simulink model "success_0516_kjh_stair_test"  (R2022b)
settings: Solver=ode45  StartTime=0.0  StopTime=15  MaxStep=0.3  RelTol=1e-3
values from neighbouring files (symbols this model uses):
  g = 9.81    [make_circle.m]
undefined symbols (not defined in the file or in its folder): fifth, first, fourth, pane, second, third, X, Y, Z
libraries: sm_lib x151, nesl_utility x13, simulink x10, slpidlib x5, Contact_Forces_Lib x2
(part 6 of 6)

== system success_0516_kjh_stair_test/right wheel ==
  Cylindrical Solid4 : sm_lib/Body Elements/Cylindrical Solid  GraphicAmbientColor=[0.15 0.15 0.15 1.0]  BasedOnType=Mass  CenterOfMass=[0 0 0]  CenterOfMassUnits=m  GraphicDiffuseColor=[0.5 0.5 0.5]  CylinderLength=150  CylinderLengthUnits=mm  CylinderRadius=5  CylinderRadiusUnits=mm  Density=2700  DensityUnits=kg/m^3  DoExposeReferenceFrame=on  GraphicEmissiveColor=[0.0 0.0 0.0 1.0]  ExportEntireGeometry=on  SerializedFrames=<Frames/>  MarkerShape=Sphere  MarkerSize=10  GraphicType=FromGeometry  InertiaType=CalculateFromGeometry  Mass=115  MassUnits=g  MomentsOfInertia=[1 1 1]  MomentsOfInertiaUnits=kg*m^2  GraphicOpacity=1.0  ProductsOfInertia=[0 0 0]  ProductsOfInertiaUnits=kg*m^2  GraphicShininess=75  GraphicSpecularColor=[0.5 0.5 0.5 1.0]  GraphicVisPropType=SimpleVisualProperties
  File Solid1 : sm_lib/Body Elements/File Solid  ExtGeomFileName=C:\Users\vbnfg\OneDrive\바탕 화면\Castone design - 복사본\tyre_ipt_2dd205d0.STEP  UnitType=FromFile  ExtGeomFileUnits=m  StepReaderType=HEX  ExportConvexHullGeometry=on  InertiaType=CalculateFromGeometry  Mass=0.12  MassUnits=kg  CenterOfMass=[0 0 0]  CenterOfMassUnits=m  MomentsOfInertia=[1 1 1]  MomentsOfInertiaUnits=kg*m^2  ProductsOfInertia=[0 0 0]  ProductsOfInertiaUnits=kg*m^2  BasedOnType=Mass  Density=2700  DensityUnits=kg/m^3  DoExposeReferenceFrame=on  SerializedFrames=<Frames/>  GraphicType=FromGeometry  MarkerShape=Sphere  MarkerSize=10  GraphicVisPropType=SimpleVisualProperties  GraphicDiffuseColor=[0.5 0.5 0.5]  GraphicSpecularColor=[0.5 0.5 0.5 1.0]  GraphicAmbientColor=[0.15 0.15 0.15 1.0]  GraphicEmissiveColor=[0.0 0.0 0.0 1.0]  GraphicShininess=75  GraphicOpacity=1.0
  File Solid7 : sm_lib/Body Elements/File Solid  ExtGeomFileName=C:\Users\vbnfg\OneDrive\바탕 화면\Castone design - 복사본\wheel.stp  UnitType=FromFile  ExtGeomFileUnits=m  StepReaderType=HEX  ExportConvexHullGeometry=on  InertiaType=CalculateFromGeometry  Mass=1.2  MassUnits=kg  CenterOfMass=[0 0 0]  CenterOfMassUnits=m  MomentsOfInertia=[1 1 1]  MomentsOfInertiaUnits=kg*m^2  ProductsOfInertia=[0 0 0]  ProductsOfInertiaUnits=kg*m^2  BasedOnType=Mass  Density=2700  DensityUnits=kg/m^3  DoExposeReferenceFrame=on  SerializedFrames=<Frames/>  GraphicType=FromGeometry  MarkerShape=Sphere  MarkerSize=10  GraphicVisPropType=SimpleVisualProperties  GraphicDiffuseColor=[0.5 0.5 0.5]  GraphicSpecularColor=[0.5 0.5 0.5 1.0]  GraphicAmbientColor=[0.15 0.15 0.15 1.0]  GraphicEmissiveColor=[0.0 0.0 0.0 1.0]  GraphicShininess=75  GraphicOpacity=1.0
  Rigid Transform22 : sm_lib/Frames and Transforms/Rigid Transform  TranslationMethod=StandardAxis  TranslationStandardOffset=-50  TranslationLengthUnit=mm  TranslationStandardAxis=+Z  TranslationCartesianOffset=[0 0 -10]  TranslationROffset=0  TranslationROffsetUnits=m  TranslationZOffset=0  TranslationZOffsetUnits=m  TranslationThetaOffset=0  TranslationThetaOffsetUnits=deg  RotationMethod=None  RotationAngleUnits=deg  RotationStandardAxis=+Z  RotationAngle=0.0  RotationArbitraryAxis=[0 0 1]  FollAlignAxisA=+X  BaseAlignAxisA=+Y  FollAlignAxisB=+Y  BaseAlignAxisB=+Z  RotationSequenceAxes=FollowerAxes  RotationSequence=XYZ  RotationSequenceAngles=[0 90 -90]  RotationSequenceAnglesUnits=deg  RotationMatrix=[1 0 0; 0 1 0; 0 0 1]  Quaternion=[1 0 0 0]
  Conn1 : PMIOPort  Side=Left
  G2 : PMIOPort  Port=2  Side=Left
  G1 : PMIOPort  Port=3  Side=Left
  connections:
  Rigid Transform22/LConn1 -- Conn1/RConn1 -- Cylindrical Solid4/RConn1
  File Solid7/RConn1 -- File Solid1/RConn1 -- Rigid Transform22/RConn1
  Cylindrical Solid4/LConn1 -- G2/RConn1
  G1/RConn1 -- File Solid1/LConn1

== system success_0516_kjh_stair_test/추진블록 ==
  Ramp : simulink/Sources/Ramp  slope=-2  start=1  InitialOutput=0
  Ramp1 : simulink/Sources/Ramp  slope=2  start=2  InitialOutput=0
  Scope1 : Scope
  Sum1 : Sum  Inputs=|+++++++
  Out1 : Outport
  wires:
  Sum1/1 -> Out1/1, Scope1/1
  Ramp/1 -> Sum1/5
  Ramp1/1 -> Sum1/6

== system success_0516_kjh_stair_test/추진블록1 ==
  In1 : Inport
  Ramp : simulink/Sources/Ramp  slope=1  start=1  InitialOutput=0
  Ramp1 : simulink/Sources/Ramp  slope=-1  start=2  InitialOutput=0
  Ramp2 : simulink/Sources/Ramp  slope=2  start=4  InitialOutput=0
  Ramp3 : simulink/Sources/Ramp  slope=-2  start=5  InitialOutput=0
  Scope1 : Scope
  Sum1 : Sum  Inputs=|++++
  Out1 : Outport
  wires:
  Sum1/1 -> Out1/1, Scope1/1
  Ramp/1 -> Sum1/1
  Ramp1/1 -> Sum1/2

== system success_0516_kjh_stair_test/추진블록2 ==
  Ramp : simulink/Sources/Ramp  slope=30  start=1  InitialOutput=0
  Ramp1 : simulink/Sources/Ramp  slope=-30  start=2  InitialOutput=0
  Ramp2 : simulink/Sources/Ramp  slope=2  start=4  InitialOutput=0
  Ramp3 : simulink/Sources/Ramp  slope=-2  start=5  InitialOutput=0
  Scope1 : Scope
  Sum1 : Sum  Inputs=|++++
  Out1 : Outport
  wires:
  Sum1/1 -> Out1/1, Scope1/1
  Ramp/1 -> Sum1/1
  Ramp1/1 -> Sum1/2
